simulink model "HGvw_non_synchronized_global"  (R2021b)
settings: Solver=VariableStepAuto  StartTime=0.0  StopTime=T  MaxStep=MaxStep  RelTol=RelTol  EnableMultiTasking=on
values from neighbouring files (symbols this model uses):
  a = 0.02    [main_global.m]
  b = 0.2    [main_global.m]
  c = -55    [main_global.m]
  d = 4    [main_global.m]
  Delta = 3    [main_global.m]
  delta0 = 5    [main_global.m]
  delta1 = 3    [main_global.m]
  Iext = 10    [main_global.m]
  J = 30    [main_global.m]
  ll = 6    [main_global.m]
  rule = 1    [main_global.m]
  stateHat0 = [zHat0;xHat0;0;3;0]    [main_global.m]
  T = 120    [main_global.m]
  tau_1 = tau_m/4    (= 6.25)    [main_global.m]
  tau_2 = tau_m/3    (= 8.33333333333)    [main_global.m]
  tau_m = 25    [main_global.m]
  x0 = [-55;-3.8]    [main_global.m]
undefined symbols (not defined in the file or in its folder): C_syst, D_syst, f_syst, g_syst
libraries: simulink x7
settings Model: Creator=pmbernar  LastModifiedBy=Pauline
settings SolverCC: AlgebraicLoopSolver=TrustRegion
settings DataIOCC: LimitDataPoints=on  ReturnWorkspaceOutputs=off
settings OptimizationCC: LifeSpan=inf
settings DebuggingCC: AllowSymbolicDim=off  PregeneratedLibrarySubsystemCodeDiagnostic=none  SFUnexpectedBacktrackingDiag=warning  SFNoUnconditionalDefaultTransitionDiag=warning  SFExecutionAtInitializationDiag=none  SFMachineParentedDataDiag=warning  ArithmeticOperatorsInVariantConditions=warning
settings ModelReferenceCC: PropagateSignalLabelsOutOfModel=off
settings SFSimCC: SimUseLocalCustomCode=off  CustomCodeUndefinedFunction=UseInterfaceOnly
settings RTWCC: RTWUseLocalCustomCode=off
settings CodeAppCC: StateflowObjectComments=on
settings GRTTargetCC: TargetLangStandard=C89/C90 (ANSI)
settings ConfigComp: CovMetricSettings=dw  CovSaveCumulativeToWorkspaceVar=on  CovSaveSingleToWorkspaceVar=on  CovExternalEMLEnable=off

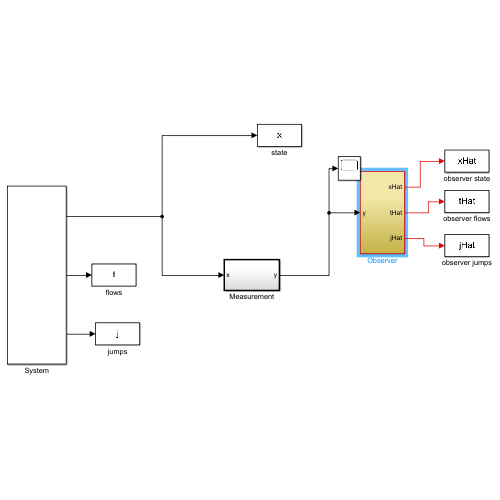
[thumbnail: Simulink's stored preview of the top-level diagram]
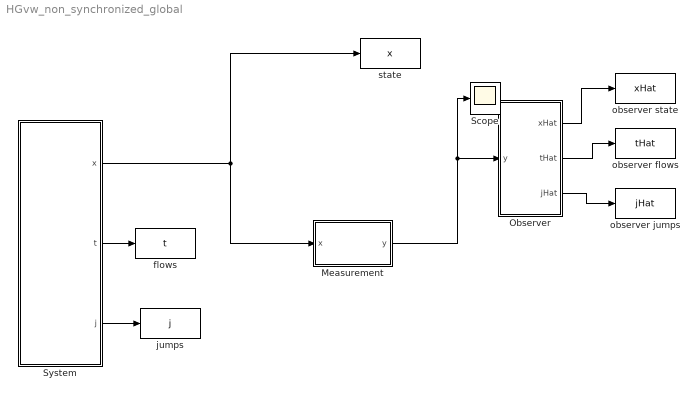
== system HGvw_non_synchronized_global ==
  Measurement : Subsystem  TreatAsAtomicUnit=on
  Observer : Subsystem  LoadFcn=set_param(gcb,'LinkStatus','none')
      settings: CopyFcn=|
      | set_param(gcb,'LinkStatus','none'),
      | set_param(gcs, 'MaxStep', 'MaxStep', 'RelTol', 'RelTol','Stop time', 'T')
  Scope : Scope
  System : Subsystem  LoadFcn=set_param(gcb,'LinkStatus','none')
      settings: CopyFcn=set_param(gcb,'LinkStatus','none')
      mask Display:
      | %image(imread('Hcalneg.jpg'))
      | %plot([5 20 20 5 5],[5 5 20 20 5])
      | %text(8,13,'HyEq_mdl')
      | color('white')
      | port_label('output', 1, 'x')
      | port_label('output', 2, 't')
      | port_label('output', 3, 'j')
  flows : ToWorkspace  VariableName=t  SampleTime=-1
  jumps : ToWorkspace  VariableName=j  SampleTime=-1
  observer flows : ToWorkspace  VariableName=tHat  SampleTime=-1
  observer jumps : ToWorkspace  VariableName=jHat  SampleTime=-1
  observer state : ToWorkspace  VariableName=xHat  SampleTime=-1
  state : ToWorkspace  VariableName=x  SampleTime=-1
  wires:
  System/2(t) -> flows/1
  System/3(j) -> jumps/1
  Measurement/1(y) -> Scope/1, Observer/1(y)
  Observer/1(xHat) -> observer state/1
  Observer/2(tHat) -> observer flows/1
  Observer/3(jHat) -> observer jumps/1
  System/1(x) -> Measurement/1(x), state/1

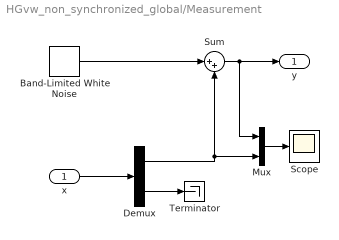
== system HGvw_non_synchronized_global/Measurement ==
  x : Inport
  Band-Limited White Noise : simulink/Sources/Band-Limited White Noise  Cov=noise  Ts=0.1  seed=[23341]
  Demux : Demux  Outputs=2
  Mux : Mux  Inputs=2
  Scope : Scope
  Sum : Sum  Inputs=|++
  Terminator : Terminator
  y : Outport  VectorParamsAs1DForOutWhenUnconnected=off
  wires:
  x/1 -> Demux/1
  Demux/2 -> Terminator/1
  Demux/1 -> Sum/2, Mux/2
  Sum/1 -> Mux/1, y/1
  Band-Limited White Noise/1 -> Sum/1
  Mux/1 -> Scope/1

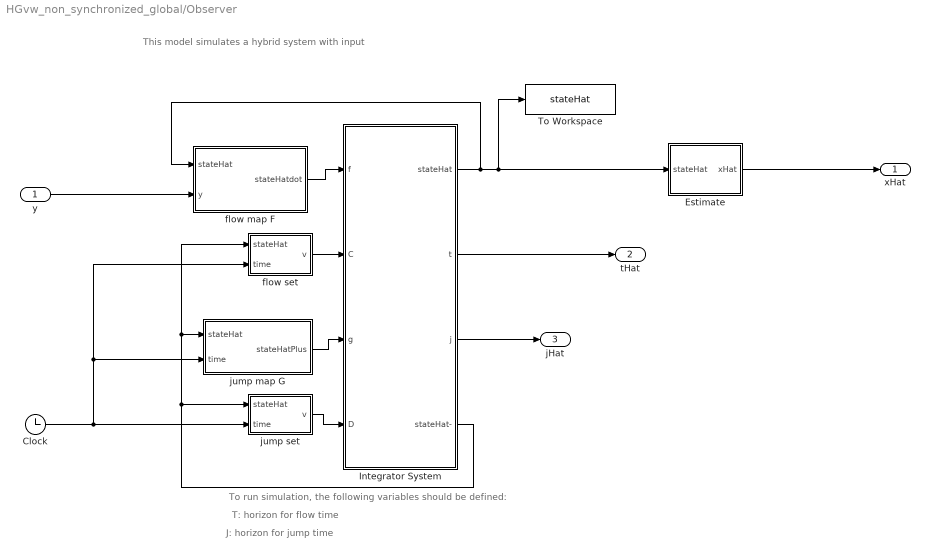
== system HGvw_non_synchronized_global/Observer ==
  note: J: horizon for jump time
  note: T: horizon for flow time
  note: To run simulation, the following variables should be defined:
  note: This model simulates a hybrid system with input
  y : Inport
  Clock : Clock
  Estimate : MATLAB Function  TreatAsAtomicUnit=on
  Integrator System : Subsystem  Priority=2  mask(Hybrid Integrator){T=T, J=J, x0=stateHat0}
      mask prompts: T "Flow Horizon"; J "Jump Horizon"; x0 "Initial Condition"
      mask help:
      | This block integrates the state of the hybrid system defined by the flow map f (first input), the flow set C (second input), the jump map g (third input) and the jump set D (fourth input).
      | Starting from the initial condition x0 (last mask parameter), the system's state x evolves continuously within the set C, according to f(x,u), but is also subject to jumps within D, according to g(x,u).
      | The block also stops the simulation when the time t is greater than the flow horizon T (first mask parameter), or when the number of jumps j is greater than the jump horizon J (second mask parameter).
      | The outputs of the blocks are respectively x(t), t, j, x(t-).
      mask Help:
      | This block integrates the state of the hybrid system defined by the flow map f (first input), the flow set C (second input), the jump map g (third input) and the jump set D (fourth input).
      | <br>
      | Starting from the initial condition x0 (last mask parameter), the system's state x evolves continuously within the set C, according to f(x,u), but is also subject to jumps within D, according to g(x,u).
      | <br>
      | The block also stops the simulation when the time t is greater than the flow horizon T (first mask parameter), or when the number of jumps j is greater than the jump horizon J (second mask parameter).
      | <br>
      | The outputs of the blocks are respectively x(t), t, j, x(t-).
      | <br>
      | You can right click on the block and "Look under mask" to see what's inside the block.
      | Finally, refer to the manual (HybridSimulator_vXX.pdf) for more detailed information on how this hybrid simulator works.
  To Workspace : ToWorkspace  VariableName=stateHat  SampleTime=-1
  flow map F : MATLAB Function  TreatAsAtomicUnit=on
  "flow set " : MATLAB Function  TreatAsAtomicUnit=on
  jump map G : MATLAB Function  Priority=2  TreatAsAtomicUnit=on
  "jump set " : MATLAB Function  TreatAsAtomicUnit=on
  xHat : Outport  VectorParamsAs1DForOutWhenUnconnected=off
  tHat : Outport  Port=2  VectorParamsAs1DForOutWhenUnconnected=off
  jHat : Outport  Port=3  VectorParamsAs1DForOutWhenUnconnected=off
  wires:
  jump map G/1(stateHatPlus) -> Integrator System/3(g)
  "jump set "/1(v) -> Integrator System/4(D)
  y/1 -> flow map F/2(y)
  Integrator System/3(j) -> jHat/1
  Integrator System/2(t) -> tHat/1
  "flow set "/1(v) -> Integrator System/2(C)
  Integrator System/1(stateHat) -> To Workspace/1, Estimate/1(stateHat), flow map F/1(stateHat)
  Integrator System/4(stateHat-) -> "flow set "/1(stateHat), jump map G/1(stateHat), "jump set "/1(stateHat)
  flow map F/1(stateHatdot) -> Integrator System/1(f)
  Estimate/1(xHat) -> xHat/1
  Clock/1 -> "flow set "/2(time), jump map G/2(time), "jump set "/2(time)

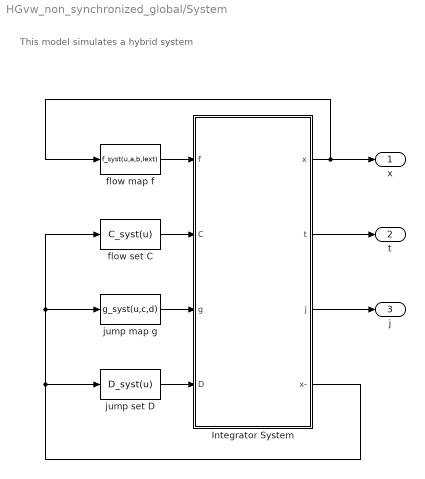
== system HGvw_non_synchronized_global/System ==
  note: This model simulates a hybrid system
  Integrator System : Subsystem  Priority=2  mask(Hybrid Integrator){T=T, J=J, x0=x0}
      mask prompts: T "Flow Horizon"; J "Jump Horizon"; x0 "Initial Condition"
      mask help:
      | This block integrates the state of the hybrid system defined by the flow map f (first input), the flow set C (second input), the jump map g (third input) and the jump set D (fourth input).
      | Starting from the initial condition x0 (last mask parameter), the system's state x evolves continuously within the set C, according to f(x,u), but is also subject to jumps within D, according to g(x,u).
      | The block also stops the simulation when the time t is greater than the flow horizon T (first mask parameter), or when the number of jumps j is greater than the jump horizon J (second mask parameter).
      | The outputs of the blocks are respectively x(t), t, j, x(t-).
      mask Help:
      | This block integrates the state of the hybrid system defined by the flow map f (first input), the flow set C (second input), the jump map g (third input) and the jump set D (fourth input).
      | <br>
      | Starting from the initial condition x0 (last mask parameter), the system's state x evolves continuously within the set C, according to f(x,u), but is also subject to jumps within D, according to g(x,u).
      | <br>
      | The block also stops the simulation when the time t is greater than the flow horizon T (first mask parameter), or when the number of jumps j is greater than the jump horizon J (second mask parameter).
      | <br>
      | The outputs of the blocks are respectively x(t), t, j, x(t-).
      | <br>
      | You can right click on the block and "Look under mask" to see what's inside the block.
      | Finally, refer to the manual (HybridSimulator_vXX.pdf) for more detailed information on how this hybrid simulator works.
  flow map f : MATLABFcn  MATLABFcn=f_syst(u,a,b,Iext)
  flow set C : MATLABFcn  MATLABFcn=C_syst(u)
  jump map g : MATLABFcn  MATLABFcn=g_syst(u,c,d)
  jump set D : MATLABFcn  MATLABFcn=D_syst(u)
  x : Outport  VectorParamsAs1DForOutWhenUnconnected=off
  t : Outport  Port=2  VectorParamsAs1DForOutWhenUnconnected=off
  j : Outport  Port=3  VectorParamsAs1DForOutWhenUnconnected=off
  wires:
  jump map g/1 -> Integrator System/3(g)
  jump set D/1 -> Integrator System/4(D)
  Integrator System/3(j) -> j/1
  Integrator System/2(t) -> t/1
  flow set C/1 -> Integrator System/2(C)
  Integrator System/1(x) -> flow map f/1, x/1
  Integrator System/4(x-) -> flow set C/1, jump map g/1, jump set D/1
  flow map f/1 -> Integrator System/1(f)

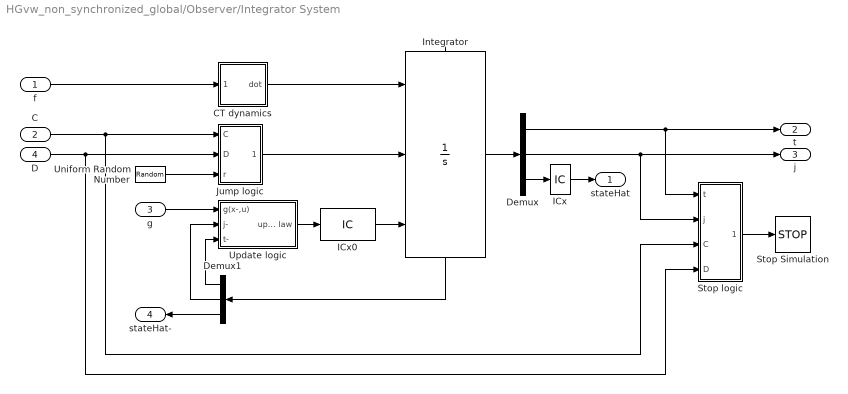
== system HGvw_non_synchronized_global/Observer/Integrator System ==
  f : Inport
  C : Inport  Port=2
  g : Inport  Port=3
  D : Inport  Port=4
  CT dynamics : Subsystem
  Demux : Demux  Outputs=[1 1 -1]
  Demux1 : Demux  Outputs=[1 1 -1]
  ICx : InitialCondition  Value=x0
  ICx0 : InitialCondition  Value=[0; 0; x0(:)]
  Integrator : Integrator  ExternalReset=level hold  InitialConditionSource=external  ShowStatePort=on  ZeroCross=off
  Jump logic : Subsystem
  Stop Simulation : Stop
  Stop logic : Subsystem
  Uniform Random Number : UniformRandomNumber  Minimum=0  Seed=abs(floor(100*rand))  SampleTime=0
  Update logic : Subsystem
  stateHat : Outport  VectorParamsAs1DForOutWhenUnconnected=off
  t : Outport  Port=2  VectorParamsAs1DForOutWhenUnconnected=off
  j : Outport  Port=3  VectorParamsAs1DForOutWhenUnconnected=off
  stateHat- : Outport  Port=4  VectorParamsAs1DForOutWhenUnconnected=off
  wires:
  ICx0/1 -> Integrator/3
  ICx/1 -> stateHat/1
  Demux/3 -> ICx/1
  Integrator/State -> Demux1/1
  Demux/2 -> j/1, Stop logic/2(j)
  Demux/1 -> t/1, Stop logic/1(t)
  Update logic/1(update law) -> ICx0/1
  CT dynamics/1(dot) -> Integrator/1
  Stop logic/1(stop) -> Stop Simulation/1
  Integrator/1 -> Demux/1
  C/1 -> Stop logic/3(C), Jump logic/1(C)
  D/1 -> Stop logic/4(D), Jump logic/2(D)
  f/1 -> CT dynamics/1(f(x,u))
  Demux1/3 -> stateHat-/1
  Jump logic/1(jump) -> Integrator/2
  Uniform Random Number/1 -> Jump logic/3(r)
  g/1 -> Update logic/1(g(x-,u))
  Demux1/1 -> Update logic/3(t-)
  Demux1/2 -> Update logic/2(j-)

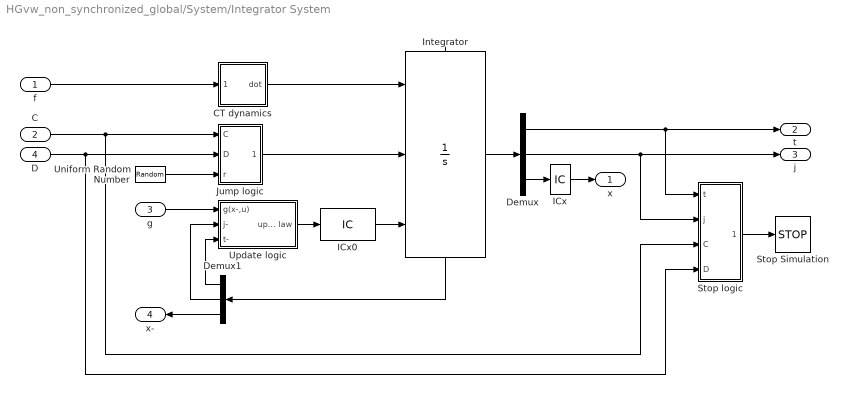
== system HGvw_non_synchronized_global/System/Integrator System ==
  f : Inport
  C : Inport  Port=2
  g : Inport  Port=3
  D : Inport  Port=4
  CT dynamics : Subsystem
  Demux : Demux  Outputs=[1 1 -1]
  Demux1 : Demux  Outputs=[1 1 -1]
  ICx : InitialCondition  Value=x0
  ICx0 : InitialCondition  Value=[0; 0; x0(:)]
  Integrator : Integrator  ExternalReset=level hold  InitialConditionSource=external  ShowStatePort=on  ZeroCross=off
  Jump logic : Subsystem
  Stop Simulation : Stop
  Stop logic : Subsystem
  Uniform Random Number : UniformRandomNumber  Minimum=0  Seed=abs(floor(100*rand))  SampleTime=0
  Update logic : Subsystem
  x : Outport  VectorParamsAs1DForOutWhenUnconnected=off
  t : Outport  Port=2  VectorParamsAs1DForOutWhenUnconnected=off
  j : Outport  Port=3  VectorParamsAs1DForOutWhenUnconnected=off
  x- : Outport  Port=4  VectorParamsAs1DForOutWhenUnconnected=off
  wires:
  ICx0/1 -> Integrator/3
  ICx/1 -> x/1
  Demux/3 -> ICx/1
  Integrator/State -> Demux1/1
  Demux/2 -> j/1, Stop logic/2(j)
  Demux/1 -> t/1, Stop logic/1(t)
  Update logic/1(update law) -> ICx0/1
  CT dynamics/1(dot) -> Integrator/1
  Stop logic/1(stop) -> Stop Simulation/1
  Integrator/1 -> Demux/1
  C/1 -> Stop logic/3(C), Jump logic/1(C)
  D/1 -> Stop logic/4(D), Jump logic/2(D)
  f/1 -> CT dynamics/1(f(x,u))
  Demux1/3 -> x-/1
  Jump logic/1(jump) -> Integrator/2
  Uniform Random Number/1 -> Jump logic/3(r)
  g/1 -> Update logic/1(g(x-,u))
  Demux1/1 -> Update logic/3(t-)
  Demux1/2 -> Update logic/2(j-)

== system HGvw_non_synchronized_global/Observer/Integrator System/CT dynamics ==
  f(x,u) : Inport
  Flows : Constant
  Jumps : Constant  Value=0
  Mux : Mux  Inputs=[1 1 -1]
  dot : Outport  VectorParamsAs1DForOutWhenUnconnected=off
  wires:
  Jumps/1 -> Mux/2
  Flows/1 -> Mux/1
  Mux/1 -> dot/1
  f(x,u)/1 -> Mux/3

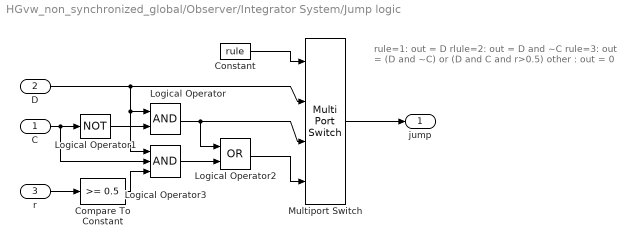
== system HGvw_non_synchronized_global/Observer/Integrator System/Jump logic ==
  note: rule=1:  out = D
      | rlule=2: out = D and ~C
      | rule=3:  out = (D and ~C)  or (D and C and r>0.5)
      | other :  out = 0
  C : Inport
  D : Inport  Port=2
  r : Inport  Port=3
  Compare To Constant : simulink/Logic and Bit Operations/Compare To Constant  relop=>=  const=0.5  OutDataTypeStr=uint8
  Constant : Constant  Value=rule
  Logical Operator : Logic  AllPortsSameDT=off  OutDataTypeStr=boolean
  Logical Operator1 : Logic  Operator=NOT  Inputs=1  AllPortsSameDT=off  OutDataTypeStr=boolean
  Logical Operator2 : Logic  Operator=OR  AllPortsSameDT=off  OutDataTypeStr=boolean
  Logical Operator3 : Logic  Inputs=3  AllPortsSameDT=off  OutDataTypeStr=boolean
  Multiport Switch : MultiPortSwitch
  jump : Outport  VectorParamsAs1DForOutWhenUnconnected=off
  wires:
  Constant/1 -> Multiport Switch/1
  D/1 -> Logical Operator3/1, Logical Operator/1, Multiport Switch/2
  r/1 -> Compare To Constant/1
  C/1 -> Logical Operator3/2, Logical Operator1/1
  Logical Operator1/1 -> Logical Operator/2
  Logical Operator/1 -> Multiport Switch/3, Logical Operator2/1
  Logical Operator2/1 -> Multiport Switch/4
  Multiport Switch/1 -> jump/1
  Compare To Constant/1 -> Logical Operator3/3
  Logical Operator3/1 -> Logical Operator2/2

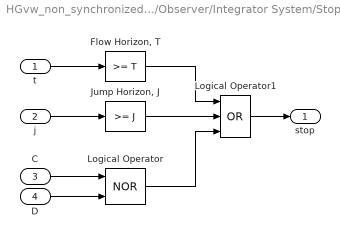
== system HGvw_non_synchronized_global/Observer/Integrator System/Stop logic ==
  t : Inport
  j : Inport  Port=2
  C : Inport  Port=3
  D : Inport  Port=4
  "Flow Horizon, T" : simulink/Logic and Bit Operations/Compare To Constant  relop=>=  const=T  OutDataTypeStr=uint8  ZeroCross=off
  "Jump Horizon, J" : simulink/Logic and Bit Operations/Compare To Constant  relop=>=  const=J  OutDataTypeStr=uint8  ZeroCross=off
  Logical Operator : Logic  Operator=NOR  AllPortsSameDT=off  OutDataTypeStr=boolean
  Logical Operator1 : Logic  Operator=OR  Inputs=3  AllPortsSameDT=off  OutDataTypeStr=boolean
  stop : Outport  VectorParamsAs1DForOutWhenUnconnected=off
  wires:
  "Flow Horizon, T"/1 -> Logical Operator1/1
  "Jump Horizon, J"/1 -> Logical Operator1/2
  Logical Operator/1 -> Logical Operator1/3
  D/1 -> Logical Operator/2
  t/1 -> "Flow Horizon, T"/1
  j/1 -> "Jump Horizon, J"/1
  C/1 -> Logical Operator/1
  Logical Operator1/1 -> stop/1

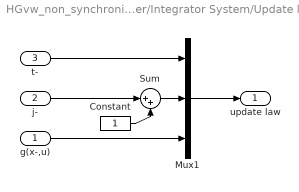
== system HGvw_non_synchronized_global/Observer/Integrator System/Update logic ==
  g(x-,u) : Inport
  j- : Inport  Port=2
  t- : Inport  Port=3
  Constant : Constant
  Mux1 : Mux  Inputs=[1 1 -1]
  Sum : Sum  Inputs=|++
  update law : Outport  VectorParamsAs1DForOutWhenUnconnected=off
  wires:
  Sum/1 -> Mux1/2
  Mux1/1 -> update law/1
  j-/1 -> Sum/1
  g(x-,u)/1 -> Mux1/3
  t-/1 -> Mux1/1
  Constant/1 -> Sum/2

== system HGvw_non_synchronized_global/System/Integrator System/CT dynamics ==
  f(x,u) : Inport
  Flows : Constant
  Jumps : Constant  Value=0
  Mux : Mux  Inputs=[1 1 -1]
  dot : Outport  VectorParamsAs1DForOutWhenUnconnected=off
  wires:
  Jumps/1 -> Mux/2
  Flows/1 -> Mux/1
  Mux/1 -> dot/1
  f(x,u)/1 -> Mux/3

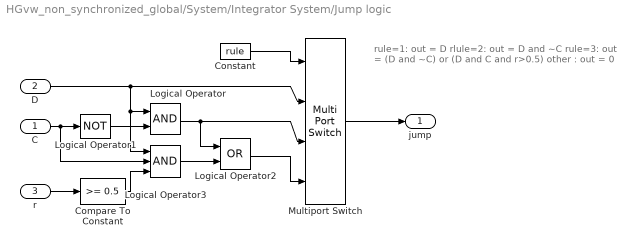
== system HGvw_non_synchronized_global/System/Integrator System/Jump logic ==
  note: rule=1:  out = D
      | rlule=2: out = D and ~C
      | rule=3:  out = (D and ~C)  or (D and C and r>0.5)
      | other :  out = 0
  C : Inport
  D : Inport  Port=2
  r : Inport  Port=3
  Compare To Constant : simulink/Logic and Bit Operations/Compare To Constant  relop=>=  const=0.5  OutDataTypeStr=uint8
  Constant : Constant  Value=rule
  Logical Operator : Logic  AllPortsSameDT=off  OutDataTypeStr=boolean
  Logical Operator1 : Logic  Operator=NOT  Inputs=1  AllPortsSameDT=off  OutDataTypeStr=boolean
  Logical Operator2 : Logic  Operator=OR  AllPortsSameDT=off  OutDataTypeStr=boolean
  Logical Operator3 : Logic  Inputs=3  AllPortsSameDT=off  OutDataTypeStr=boolean
  Multiport Switch : MultiPortSwitch
  jump : Outport  VectorParamsAs1DForOutWhenUnconnected=off
  wires:
  Constant/1 -> Multiport Switch/1
  D/1 -> Logical Operator3/1, Logical Operator/1, Multiport Switch/2
  r/1 -> Compare To Constant/1
  C/1 -> Logical Operator3/2, Logical Operator1/1
  Logical Operator1/1 -> Logical Operator/2
  Logical Operator/1 -> Multiport Switch/3, Logical Operator2/1
  Logical Operator2/1 -> Multiport Switch/4
  Multiport Switch/1 -> jump/1
  Compare To Constant/1 -> Logical Operator3/3
  Logical Operator3/1 -> Logical Operator2/2

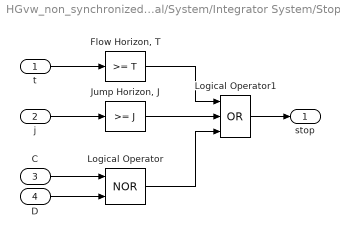
== system HGvw_non_synchronized_global/System/Integrator System/Stop logic ==
  t : Inport
  j : Inport  Port=2
  C : Inport  Port=3
  D : Inport  Port=4
  "Flow Horizon, T" : simulink/Logic and Bit Operations/Compare To Constant  relop=>=  const=T  OutDataTypeStr=uint8  ZeroCross=off
  "Jump Horizon, J" : simulink/Logic and Bit Operations/Compare To Constant  relop=>=  const=J  OutDataTypeStr=uint8  ZeroCross=off
  Logical Operator : Logic  Operator=NOR  AllPortsSameDT=off  OutDataTypeStr=boolean
  Logical Operator1 : Logic  Operator=OR  Inputs=3  AllPortsSameDT=off  OutDataTypeStr=boolean
  stop : Outport  VectorParamsAs1DForOutWhenUnconnected=off
  wires:
  "Flow Horizon, T"/1 -> Logical Operator1/1
  "Jump Horizon, J"/1 -> Logical Operator1/2
  Logical Operator/1 -> Logical Operator1/3
  D/1 -> Logical Operator/2
  t/1 -> "Flow Horizon, T"/1
  j/1 -> "Jump Horizon, J"/1
  C/1 -> Logical Operator/1
  Logical Operator1/1 -> stop/1

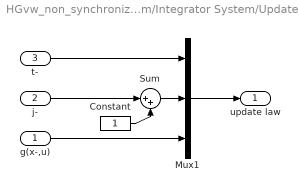
== system HGvw_non_synchronized_global/System/Integrator System/Update logic ==
  g(x-,u) : Inport
  j- : Inport  Port=2
  t- : Inport  Port=3
  Constant : Constant
  Mux1 : Mux  Inputs=[1 1 -1]
  Sum : Sum  Inputs=|++
  update law : Outport  VectorParamsAs1DForOutWhenUnconnected=off
  wires:
  Sum/1 -> Mux1/2
  Mux1/1 -> update law/1
  j-/1 -> Sum/1
  g(x-,u)/1 -> Mux1/3
  t-/1 -> Mux1/1
  Constant/1 -> Sum/2

== matlab function HGvw_non_synchronized_global/Observer/flow map F ==
  data: stateHat input; stateHatdot output; y input; ll parameter; a parameter; b parameter; Iext parameter
function stateHatdot = F(stateHat, y,ll,a, b, Iext)

zHat = stateHat(1:2);
chi = stateHat(3:4);
% tau = stateHat(5);
q = stateHat(6);
% warn = stateHat(7);

if (q==2 || q==3)

    % high gain observer
    Ac = [0,1;0,0];
    Lc = [ll;ll^2];

    xHat = compute_x(zHat,Iext);

    % bornes pour saturation |v|<80, |w|<10, |z2|<820 ->  |phi|<9300

    phi = (0.04*2*xHat(1)+5)*zHat(2)-a*(b*xHat(1)-xHat(2));
    phi = min(max(phi,-9000),9000);
    Bc = [0;1];

    zHatdot = Ac*zHat+Bc*phi+Lc*(y-zHat(1));
    
    chidot = zeros(2,1);
    
    taudot = 0;
    
elseif q==1
    
    zHatdot =  zeros(2,1);
    chidot = [0.04*chi(1)^2+5*chi(1)+140-chi(2)+Iext;a*(b*chi(1)-chi(2))];
    taudot = 0;
    
else
    zHatdot =  zeros(2,1);
    chidot = [0.04*chi(1)^2+5*chi(1)+140-chi(2)+Iext;a*(b*chi(1)-chi(2))];
    taudot = 1;
end

qdot = 0;
warndot = 0;

stateHatdot = [zHatdot;chidot;taudot;qdot;warndot];

== matlab function HGvw_non_synchronized_global/Observer/Estimate ==
  data: stateHat input; xHat output; Iext parameter
function xHat = fcn(stateHat,Iext)

zHat = stateHat(1:2);
chi = stateHat(3:4);
tau = stateHat(5);
q = stateHat(6);

if q==2 || q==3
    xHat = compute_x(zHat,Iext);
else
    xHat = chi;
end

== matlab function HGvw_non_synchronized_global/Observer/flow set  ==
  data: stateHat input; v output; Iext parameter; time input; delta1 parameter; delta0 parameter; Delta parameter; tau_1 parameter; tau_2 parameter; tau_m parameter
function v  = Chat(stateHat,Iext,time, delta1, delta0, Delta, tau_1, tau_2, tau_m) 

zHat = stateHat(1:2);
chi = stateHat(3:4);
tau = stateHat(5);
q = stateHat(6);
warn = stateHat(7);

xHat = compute_x(zHat,Iext);
xHat(1) = min([xHat(1),30]); % projection on C \cup D
test_C_delta1 = (xHat(1)<=30-delta1);
test_D_delta0 = (chi(1)>=30-delta0 && chi(1)<=30);

if (q==3 && time<=tau_m && warn==1)  % flow condition
    v = 1; % report flow
elseif (q==3 && time<=tau_1)  % flow condition
     v = 1; % report flow
elseif (q==3 && time<=tau_m && test_C_delta1)   % flow condition
    v = 1; % report flow
elseif (q==2 && test_C_delta1)  % flow condition
    v = 1;  % report flow
elseif (q==1 &&  test_D_delta0)  % flow condition
    v = 1;  % report flow
elseif (q==0 && tau<=Delta)  % flow condition
    v = 1;  % report flow
else
    v = 0;   % do not report flow
end

== matlab function HGvw_non_synchronized_global/Observer/jump map G ==
  data: stateHat input; time input; stateHatPlus output; d parameter; Iext parameter; c parameter; delta1 parameter; tau_1 parameter; tau_2 parameter
function stateHatPlus = G(stateHat,time,d,Iext, c,delta1,tau_1, tau_2)

zHat = stateHat(1:2);
chi = stateHat(3:4);
% tau = stateHat(5);
q = stateHat(6);
% warn = stateHat(7);

xHat = compute_x(zHat,Iext);
xHat(1) = min([xHat(1),30]); % projection on C\cup D
test_D_delta1 = (xHat(1)<=30-delta1);

if (q==3 && time>=tau_1 && time<=tau_2) 
    stateHatPlus = stateHat;
    stateHatPlus(7) = 1; % set warning state to 1
elseif (q==3 && test_D_delta1)
    stateHatPlus = stateHat;
    stateHatPlus(6) = 2; % switch to local hybrid observer with mode 2
    stateHatPlus(7) = 0; % set warning state (back) to 0
elseif (q==3)
    stateHatPlus = [zHat;xHat;0;1;0];% switch to local hybrid observer with mode 1
elseif q==2
    stateHatPlus = [zHat;xHat;0;1;0];
elseif q==1
    stateHatPlus = [zHat;c;chi(2)+d;0;0;0];
else
    chi(1) = min([chi(1),30]); % projection on C\cup D
    stateHatPlus = [compute_z(chi,Iext);chi;0;2;0];
end

== matlab function HGvw_non_synchronized_global/Observer/jump set  ==
  data: v output; stateHat input; time input; Iext parameter; delta1 parameter; delta0 parameter; Delta parameter; tau_m parameter; tau_1 parameter; tau_2 parameter
function v  = Dhat(stateHat,time,Iext, delta1, delta0, Delta, tau_m,tau_1, tau_2) 

zHat = stateHat(1:2);
chi = stateHat(3:4);
tau = stateHat(5);
q = stateHat(6);
warn = stateHat(7);

xHat = compute_x(zHat,Iext);
test_C_delta0 = (chi(1)<=30-delta0);
test_D_delta1 = (xHat(1)>=30-delta1);
test_D = (chi(1)>=30);

if (q==3 && time>=tau_1 && time<=tau_2 && test_D_delta1 && warn==0) 
    v = 1;
elseif (q==3 && time>=tau_2 && test_D_delta1 && warn == 0)
    v = 1;
elseif (q==3 && time >=tau_m)
    v=1;
elseif (q==2 && test_D_delta1)  % jump condition
    v = 1;  % report jump
elseif (q==1 && test_D)  % jump condition
    v = 1;  % report jump
elseif (q==0 && test_C_delta0 && tau>=Delta)  % jump condition
    v = 1;  % report jump
else
    v = 0;   % do not report jump
end
